simulink model "scheme5"  (R2024a)
settings: Solver=VariableStepAuto  StartTime=0.0  StopTime=100  RelTol=1e-6
values from neighbouring files (symbols this model uses):
  func = sin_node(A, 0.25)    [main.m]
undefined symbols (not defined in the file or in its folder): ki, kp
settings Model: Creator=alexivanov  LastModifiedBy=alexivanov

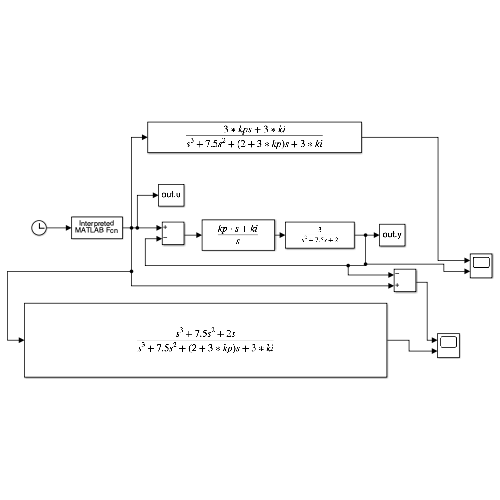
[thumbnail: Simulink's stored preview of the top-level diagram]
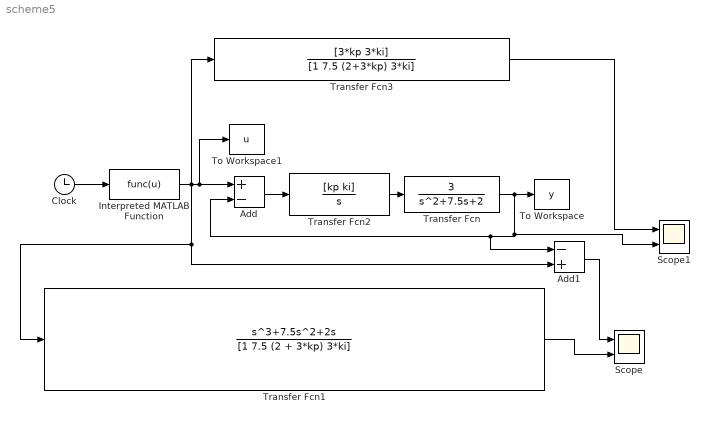
== system scheme5 ==
  Add : Sum  Inputs=+-
  Add1 : Sum  Inputs=-+
  Clock : Clock
  Interpreted MATLAB Function : MATLABFcn  MATLABFcn=func(u)
  Scope : Scope  NumInputPorts=2
  Scope1 : Scope  NumInputPorts=2
  To Workspace : ToWorkspace  VariableName=y  SaveFormat=Timeseries  SampleTime=-1
  To Workspace1 : ToWorkspace  VariableName=u  SaveFormat=Timeseries  SampleTime=-1
  Transfer Fcn : TransferFcn  Numerator=[3]  Denominator=[1 7.5 2]
  Transfer Fcn1 : TransferFcn  Numerator=[1 7.5 2 0]  Denominator=[1 7.5 (2 + 3*kp) 3*ki]
  Transfer Fcn2 : TransferFcn  Numerator=[kp ki]  Denominator=[1 0]
  Transfer Fcn3 : TransferFcn  Numerator=[3*kp 3*ki]  Denominator=[1 7.5 (2+3*kp) 3*ki]
  wires:
  Clock/1 -> Interpreted MATLAB Function/1
  Transfer Fcn2/1 -> Transfer Fcn/1
  Add/1 -> Transfer Fcn2/1
  Interpreted MATLAB Function/1 -> Transfer Fcn3/1, Add1/2, Transfer Fcn1/1, To Workspace1/1, Add/1
  Transfer Fcn/1 -> Add1/1, Add/2, Scope1/2, To Workspace/1
  Transfer Fcn1/1 -> Scope/2
  Add1/1 -> Scope/1
  Transfer Fcn3/1 -> Scope1/1
